simulink model "PTTransmCU"  (R2022b)
settings: Solver=ode45  StartTime=0.0  StopTime=inf  RelTol=1e-3  EnableMultiTasking=on
libraries: simulink x2, CarMaker4SL x1
(part 4 of 5)

== system PTTransmCU/CarMaker/IPG Vehicle/PowerTrain/TCU Example/PTTransmCU_In/CreateBus TCU GearboxIn8 ==
  In : Inport
  BusCreator : BusCreator  Inputs=23
  Demux : Demux  Outputs=23
      settings: DisplayOption=none
  Out : Outport  VectorParamsAs1DForOutWhenUnconnected=off
  wires:
  Demux/23 -> BusCreator/23  "TCU GearboxIn8 Clutch_dis i_TrqIn2Out"
  Demux/22 -> BusCreator/22  "TCU GearboxIn8 Clutch_dis Trq_out_trg"
  Demux/21 -> BusCreator/21  "TCU GearboxIn8 Clutch_dis Trq_out"
  Demux/20 -> BusCreator/20  "TCU GearboxIn8 Clutch_dis Trq_in"
  Demux/19 -> BusCreator/19  "TCU GearboxIn8 Clutch_dis rotv_out_trg"
  Demux/18 -> BusCreator/18  "TCU GearboxIn8 Clutch_dis rotv_out"
  Demux/17 -> BusCreator/17  "TCU GearboxIn8 Clutch_dis rotv_in"
  Demux/16 -> BusCreator/16  "TCU GearboxIn8 Clutch i_TrqIn2Out"
  Demux/15 -> BusCreator/15  "TCU GearboxIn8 Clutch Trq_out_trg"
  Demux/14 -> BusCreator/14  "TCU GearboxIn8 Clutch Trq_out"
  Demux/13 -> BusCreator/13  "TCU GearboxIn8 Clutch Trq_in"
  Demux/12 -> BusCreator/12  "TCU GearboxIn8 Clutch rotv_out_trg"
  Demux/11 -> BusCreator/11  "TCU GearboxIn8 Clutch rotv_out"
  Demux/10 -> BusCreator/10  "TCU GearboxIn8 Clutch rotv_in"
  Demux/9 -> BusCreator/9  "TCU GearboxIn8 Trq_out_trg"
  Demux/8 -> BusCreator/8  "TCU GearboxIn8 Trq_out"
  Demux/7 -> BusCreator/7  "TCU GearboxIn8 Trq_in"
  Demux/6 -> BusCreator/6  "TCU GearboxIn8 rotv_out"
  Demux/5 -> BusCreator/5  "TCU GearboxIn8 rotv_in_trg"
  Demux/4 -> BusCreator/4  "TCU GearboxIn8 rotv_in"
  Demux/3 -> BusCreator/3  "TCU GearboxIn8 i"
  Demux/2 -> BusCreator/2  "TCU GearboxIn8 GearNo_dis"
  Demux/1 -> BusCreator/1  "TCU GearboxIn8 GearNo"
  BusCreator/1 -> Out/1
  In/1 -> Demux/1

== system PTTransmCU/CarMaker/IPG Vehicle/PowerTrain/TCU Example/PTTransmCU_In/CreateBus TCU GearboxIn9 ==
  In : Inport
  BusCreator : BusCreator  Inputs=23
  Demux : Demux  Outputs=23
      settings: DisplayOption=none
  Out : Outport  VectorParamsAs1DForOutWhenUnconnected=off
  wires:
  Demux/23 -> BusCreator/23  "TCU GearboxIn9 Clutch_dis i_TrqIn2Out"
  Demux/22 -> BusCreator/22  "TCU GearboxIn9 Clutch_dis Trq_out_trg"
  Demux/21 -> BusCreator/21  "TCU GearboxIn9 Clutch_dis Trq_out"
  Demux/20 -> BusCreator/20  "TCU GearboxIn9 Clutch_dis Trq_in"
  Demux/19 -> BusCreator/19  "TCU GearboxIn9 Clutch_dis rotv_out_trg"
  Demux/18 -> BusCreator/18  "TCU GearboxIn9 Clutch_dis rotv_out"
  Demux/17 -> BusCreator/17  "TCU GearboxIn9 Clutch_dis rotv_in"
  Demux/16 -> BusCreator/16  "TCU GearboxIn9 Clutch i_TrqIn2Out"
  Demux/15 -> BusCreator/15  "TCU GearboxIn9 Clutch Trq_out_trg"
  Demux/14 -> BusCreator/14  "TCU GearboxIn9 Clutch Trq_out"
  Demux/13 -> BusCreator/13  "TCU GearboxIn9 Clutch Trq_in"
  Demux/12 -> BusCreator/12  "TCU GearboxIn9 Clutch rotv_out_trg"
  Demux/11 -> BusCreator/11  "TCU GearboxIn9 Clutch rotv_out"
  Demux/10 -> BusCreator/10  "TCU GearboxIn9 Clutch rotv_in"
  Demux/9 -> BusCreator/9  "TCU GearboxIn9 Trq_out_trg"
  Demux/8 -> BusCreator/8  "TCU GearboxIn9 Trq_out"
  Demux/7 -> BusCreator/7  "TCU GearboxIn9 Trq_in"
  Demux/6 -> BusCreator/6  "TCU GearboxIn9 rotv_out"
  Demux/5 -> BusCreator/5  "TCU GearboxIn9 rotv_in_trg"
  Demux/4 -> BusCreator/4  "TCU GearboxIn9 rotv_in"
  Demux/3 -> BusCreator/3  "TCU GearboxIn9 i"
  Demux/2 -> BusCreator/2  "TCU GearboxIn9 GearNo_dis"
  Demux/1 -> BusCreator/1  "TCU GearboxIn9 GearNo"
  BusCreator/1 -> Out/1
  In/1 -> Demux/1

== system PTTransmCU/CarMaker/IPG Vehicle/PowerTrain/TCU Example/PTTransmCU_In/CreateBus TCU GearboxOut0 ==
  In : Inport
  BusCreator : BusCreator  Inputs=6
  Demux : Demux  Outputs=6
      settings: DisplayOption=none
  Out : Outport  VectorParamsAs1DForOutWhenUnconnected=off
  wires:
  Demux/6 -> BusCreator/6  "TCU GearboxOut0 Clutch_dis Pos"
  Demux/5 -> BusCreator/5  "TCU GearboxOut0 Clutch Pos"
  Demux/4 -> BusCreator/4  "TCU GearboxOut0 i_trg"
  Demux/3 -> BusCreator/3  "TCU GearboxOut0 set_ParkBrake"
  Demux/2 -> BusCreator/2  "TCU GearboxOut0 GearNoTrg_dis"
  Demux/1 -> BusCreator/1  "TCU GearboxOut0 GearNoTrg"
  BusCreator/1 -> Out/1
  In/1 -> Demux/1

== system PTTransmCU/CarMaker/IPG Vehicle/PowerTrain/TCU Example/PTTransmCU_In/CreateBus TCU GearboxOut1 ==
  In : Inport
  BusCreator : BusCreator  Inputs=6
  Demux : Demux  Outputs=6
      settings: DisplayOption=none
  Out : Outport  VectorParamsAs1DForOutWhenUnconnected=off
  wires:
  Demux/6 -> BusCreator/6  "TCU GearboxOut1 Clutch_dis Pos"
  Demux/5 -> BusCreator/5  "TCU GearboxOut1 Clutch Pos"
  Demux/4 -> BusCreator/4  "TCU GearboxOut1 i_trg"
  Demux/3 -> BusCreator/3  "TCU GearboxOut1 set_ParkBrake"
  Demux/2 -> BusCreator/2  "TCU GearboxOut1 GearNoTrg_dis"
  Demux/1 -> BusCreator/1  "TCU GearboxOut1 GearNoTrg"
  BusCreator/1 -> Out/1
  In/1 -> Demux/1

== system PTTransmCU/CarMaker/IPG Vehicle/PowerTrain/TCU Example/PTTransmCU_In/CreateBus TCU GearboxOut10 ==
  In : Inport
  BusCreator : BusCreator  Inputs=6
  Demux : Demux  Outputs=6
      settings: DisplayOption=none
  Out : Outport  VectorParamsAs1DForOutWhenUnconnected=off
  wires:
  Demux/6 -> BusCreator/6  "TCU GearboxOut10 Clutch_dis Pos"
  Demux/5 -> BusCreator/5  "TCU GearboxOut10 Clutch Pos"
  Demux/4 -> BusCreator/4  "TCU GearboxOut10 i_trg"
  Demux/3 -> BusCreator/3  "TCU GearboxOut10 set_ParkBrake"
  Demux/2 -> BusCreator/2  "TCU GearboxOut10 GearNoTrg_dis"
  Demux/1 -> BusCreator/1  "TCU GearboxOut10 GearNoTrg"
  BusCreator/1 -> Out/1
  In/1 -> Demux/1

== system PTTransmCU/CarMaker/IPG Vehicle/PowerTrain/TCU Example/PTTransmCU_In/CreateBus TCU GearboxOut11 ==
  In : Inport
  BusCreator : BusCreator  Inputs=6
  Demux : Demux  Outputs=6
      settings: DisplayOption=none
  Out : Outport  VectorParamsAs1DForOutWhenUnconnected=off
  wires:
  Demux/6 -> BusCreator/6  "TCU GearboxOut11 Clutch_dis Pos"
  Demux/5 -> BusCreator/5  "TCU GearboxOut11 Clutch Pos"
  Demux/4 -> BusCreator/4  "TCU GearboxOut11 i_trg"
  Demux/3 -> BusCreator/3  "TCU GearboxOut11 set_ParkBrake"
  Demux/2 -> BusCreator/2  "TCU GearboxOut11 GearNoTrg_dis"
  Demux/1 -> BusCreator/1  "TCU GearboxOut11 GearNoTrg"
  BusCreator/1 -> Out/1
  In/1 -> Demux/1

== system PTTransmCU/CarMaker/IPG Vehicle/PowerTrain/TCU Example/PTTransmCU_In/CreateBus TCU GearboxOut2 ==
  In : Inport
  BusCreator : BusCreator  Inputs=6
  Demux : Demux  Outputs=6
      settings: DisplayOption=none
  Out : Outport  VectorParamsAs1DForOutWhenUnconnected=off
  wires:
  Demux/6 -> BusCreator/6  "TCU GearboxOut2 Clutch_dis Pos"
  Demux/5 -> BusCreator/5  "TCU GearboxOut2 Clutch Pos"
  Demux/4 -> BusCreator/4  "TCU GearboxOut2 i_trg"
  Demux/3 -> BusCreator/3  "TCU GearboxOut2 set_ParkBrake"
  Demux/2 -> BusCreator/2  "TCU GearboxOut2 GearNoTrg_dis"
  Demux/1 -> BusCreator/1  "TCU GearboxOut2 GearNoTrg"
  BusCreator/1 -> Out/1
  In/1 -> Demux/1

== system PTTransmCU/CarMaker/IPG Vehicle/PowerTrain/TCU Example/PTTransmCU_In/CreateBus TCU GearboxOut3 ==
  In : Inport
  BusCreator : BusCreator  Inputs=6
  Demux : Demux  Outputs=6
      settings: DisplayOption=none
  Out : Outport  VectorParamsAs1DForOutWhenUnconnected=off
  wires:
  Demux/6 -> BusCreator/6  "TCU GearboxOut3 Clutch_dis Pos"
  Demux/5 -> BusCreator/5  "TCU GearboxOut3 Clutch Pos"
  Demux/4 -> BusCreator/4  "TCU GearboxOut3 i_trg"
  Demux/3 -> BusCreator/3  "TCU GearboxOut3 set_ParkBrake"
  Demux/2 -> BusCreator/2  "TCU GearboxOut3 GearNoTrg_dis"
  Demux/1 -> BusCreator/1  "TCU GearboxOut3 GearNoTrg"
  BusCreator/1 -> Out/1
  In/1 -> Demux/1

== system PTTransmCU/CarMaker/IPG Vehicle/PowerTrain/TCU Example/PTTransmCU_In/CreateBus TCU GearboxOut4 ==
  In : Inport
  BusCreator : BusCreator  Inputs=6
  Demux : Demux  Outputs=6
      settings: DisplayOption=none
  Out : Outport  VectorParamsAs1DForOutWhenUnconnected=off
  wires:
  Demux/6 -> BusCreator/6  "TCU GearboxOut4 Clutch_dis Pos"
  Demux/5 -> BusCreator/5  "TCU GearboxOut4 Clutch Pos"
  Demux/4 -> BusCreator/4  "TCU GearboxOut4 i_trg"
  Demux/3 -> BusCreator/3  "TCU GearboxOut4 set_ParkBrake"
  Demux/2 -> BusCreator/2  "TCU GearboxOut4 GearNoTrg_dis"
  Demux/1 -> BusCreator/1  "TCU GearboxOut4 GearNoTrg"
  BusCreator/1 -> Out/1
  In/1 -> Demux/1

== system PTTransmCU/CarMaker/IPG Vehicle/PowerTrain/TCU Example/PTTransmCU_In/CreateBus TCU GearboxOut5 ==
  In : Inport
  BusCreator : BusCreator  Inputs=6
  Demux : Demux  Outputs=6
      settings: DisplayOption=none
  Out : Outport  VectorParamsAs1DForOutWhenUnconnected=off
  wires:
  Demux/6 -> BusCreator/6  "TCU GearboxOut5 Clutch_dis Pos"
  Demux/5 -> BusCreator/5  "TCU GearboxOut5 Clutch Pos"
  Demux/4 -> BusCreator/4  "TCU GearboxOut5 i_trg"
  Demux/3 -> BusCreator/3  "TCU GearboxOut5 set_ParkBrake"
  Demux/2 -> BusCreator/2  "TCU GearboxOut5 GearNoTrg_dis"
  Demux/1 -> BusCreator/1  "TCU GearboxOut5 GearNoTrg"
  BusCreator/1 -> Out/1
  In/1 -> Demux/1

== system PTTransmCU/CarMaker/IPG Vehicle/PowerTrain/TCU Example/PTTransmCU_In/CreateBus TCU GearboxOut6 ==
  In : Inport
  BusCreator : BusCreator  Inputs=6
  Demux : Demux  Outputs=6
      settings: DisplayOption=none
  Out : Outport  VectorParamsAs1DForOutWhenUnconnected=off
  wires:
  Demux/6 -> BusCreator/6  "TCU GearboxOut6 Clutch_dis Pos"
  Demux/5 -> BusCreator/5  "TCU GearboxOut6 Clutch Pos"
  Demux/4 -> BusCreator/4  "TCU GearboxOut6 i_trg"
  Demux/3 -> BusCreator/3  "TCU GearboxOut6 set_ParkBrake"
  Demux/2 -> BusCreator/2  "TCU GearboxOut6 GearNoTrg_dis"
  Demux/1 -> BusCreator/1  "TCU GearboxOut6 GearNoTrg"
  BusCreator/1 -> Out/1
  In/1 -> Demux/1

== system PTTransmCU/CarMaker/IPG Vehicle/PowerTrain/TCU Example/PTTransmCU_In/CreateBus TCU GearboxOut7 ==
  In : Inport
  BusCreator : BusCreator  Inputs=6
  Demux : Demux  Outputs=6
      settings: DisplayOption=none
  Out : Outport  VectorParamsAs1DForOutWhenUnconnected=off
  wires:
  Demux/6 -> BusCreator/6  "TCU GearboxOut7 Clutch_dis Pos"
  Demux/5 -> BusCreator/5  "TCU GearboxOut7 Clutch Pos"
  Demux/4 -> BusCreator/4  "TCU GearboxOut7 i_trg"
  Demux/3 -> BusCreator/3  "TCU GearboxOut7 set_ParkBrake"
  Demux/2 -> BusCreator/2  "TCU GearboxOut7 GearNoTrg_dis"
  Demux/1 -> BusCreator/1  "TCU GearboxOut7 GearNoTrg"
  BusCreator/1 -> Out/1
  In/1 -> Demux/1

== system PTTransmCU/CarMaker/IPG Vehicle/PowerTrain/TCU Example/PTTransmCU_In/CreateBus TCU GearboxOut8 ==
  In : Inport
  BusCreator : BusCreator  Inputs=6
  Demux : Demux  Outputs=6
      settings: DisplayOption=none
  Out : Outport  VectorParamsAs1DForOutWhenUnconnected=off
  wires:
  Demux/6 -> BusCreator/6  "TCU GearboxOut8 Clutch_dis Pos"
  Demux/5 -> BusCreator/5  "TCU GearboxOut8 Clutch Pos"
  Demux/4 -> BusCreator/4  "TCU GearboxOut8 i_trg"
  Demux/3 -> BusCreator/3  "TCU GearboxOut8 set_ParkBrake"
  Demux/2 -> BusCreator/2  "TCU GearboxOut8 GearNoTrg_dis"
  Demux/1 -> BusCreator/1  "TCU GearboxOut8 GearNoTrg"
  BusCreator/1 -> Out/1
  In/1 -> Demux/1

== system PTTransmCU/CarMaker/IPG Vehicle/PowerTrain/TCU Example/PTTransmCU_In/CreateBus TCU GearboxOut9 ==
  In : Inport
  BusCreator : BusCreator  Inputs=6
  Demux : Demux  Outputs=6
      settings: DisplayOption=none
  Out : Outport  VectorParamsAs1DForOutWhenUnconnected=off
  wires:
  Demux/6 -> BusCreator/6  "TCU GearboxOut9 Clutch_dis Pos"
  Demux/5 -> BusCreator/5  "TCU GearboxOut9 Clutch Pos"
  Demux/4 -> BusCreator/4  "TCU GearboxOut9 i_trg"
  Demux/3 -> BusCreator/3  "TCU GearboxOut9 set_ParkBrake"
  Demux/2 -> BusCreator/2  "TCU GearboxOut9 GearNoTrg_dis"
  Demux/1 -> BusCreator/1  "TCU GearboxOut9 GearNoTrg"
  BusCreator/1 -> Out/1
  In/1 -> Demux/1

== system PTTransmCU/CarMaker/IPG Vehicle/PowerTrain/TCU Example/PTTransmCU_In/CreateBus TCU Input ==
  In : Inport
  BusCreator : BusCreator  Inputs=3
  Demux : Demux  Outputs=3
      settings: DisplayOption=none
  Out : Outport  VectorParamsAs1DForOutWhenUnconnected=off
  wires:
  Demux/3 -> BusCreator/3  "TCU SelectorCtrl"
  Demux/2 -> BusCreator/2  "TCU Load"
  Demux/1 -> BusCreator/1  "TCU Ignition"
  BusCreator/1 -> Out/1
  In/1 -> Demux/1

== system PTTransmCU/CarMaker/IPG Vehicle/PowerTrain/TCU Example/PTTransmCU_In/CreateBus TCU_Cfg Gearbox0 ==
  In : Inport
  BusCreator : BusCreator  Inputs=38
  Demux : Demux  Outputs=38
      settings: DisplayOption=none
  Out : Outport  VectorParamsAs1DForOutWhenUnconnected=off
  wires:
  Demux/38 -> BusCreator/38  "TCU_Cfg Gearbox0 iBGear16"
  Demux/37 -> BusCreator/37  "TCU_Cfg Gearbox0 iBGear15"
  Demux/36 -> BusCreator/36  "TCU_Cfg Gearbox0 iBGear14"
  Demux/35 -> BusCreator/35  "TCU_Cfg Gearbox0 iBGear13"
  Demux/34 -> BusCreator/34  "TCU_Cfg Gearbox0 iBGear12"
  Demux/33 -> BusCreator/33  "TCU_Cfg Gearbox0 iBGear11"
  Demux/32 -> BusCreator/32  "TCU_Cfg Gearbox0 iBGear10"
  Demux/31 -> BusCreator/31  "TCU_Cfg Gearbox0 iBGear9"
  Demux/30 -> BusCreator/30  "TCU_Cfg Gearbox0 iBGear8"
  Demux/29 -> BusCreator/29  "TCU_Cfg Gearbox0 iBGear7"
  Demux/28 -> BusCreator/28  "TCU_Cfg Gearbox0 iBGear6"
  Demux/27 -> BusCreator/27  "TCU_Cfg Gearbox0 iBGear5"
  Demux/26 -> BusCreator/26  "TCU_Cfg Gearbox0 iBGear4"
  Demux/25 -> BusCreator/25  "TCU_Cfg Gearbox0 iBGear3"
  Demux/24 -> BusCreator/24  "TCU_Cfg Gearbox0 iBGear2"
  Demux/23 -> BusCreator/23  "TCU_Cfg Gearbox0 iBGear1"
  Demux/22 -> BusCreator/22  "TCU_Cfg Gearbox0 iBGear0"
  Demux/21 -> BusCreator/21  "TCU_Cfg Gearbox0 nBGears"
  Demux/20 -> BusCreator/20  "TCU_Cfg Gearbox0 iFGear16"
  Demux/19 -> BusCreator/19  "TCU_Cfg Gearbox0 iFGear15"
  Demux/18 -> BusCreator/18  "TCU_Cfg Gearbox0 iFGear14"
  Demux/17 -> BusCreator/17  "TCU_Cfg Gearbox0 iFGear13"
  Demux/16 -> BusCreator/16  "TCU_Cfg Gearbox0 iFGear12"
  Demux/15 -> BusCreator/15  "TCU_Cfg Gearbox0 iFGear11"
  Demux/14 -> BusCreator/14  "TCU_Cfg Gearbox0 iFGear10"
  Demux/13 -> BusCreator/13  "TCU_Cfg Gearbox0 iFGear9"
  Demux/12 -> BusCreator/12  "TCU_Cfg Gearbox0 iFGear8"
  Demux/11 -> BusCreator/11  "TCU_Cfg Gearbox0 iFGear7"
  Demux/10 -> BusCreator/10  "TCU_Cfg Gearbox0 iFGear6"
  Demux/9 -> BusCreator/9  "TCU_Cfg Gearbox0 iFGear5"
  Demux/8 -> BusCreator/8  "TCU_Cfg Gearbox0 iFGear4"
  Demux/7 -> BusCreator/7  "TCU_Cfg Gearbox0 iFGear3"
  Demux/6 -> BusCreator/6  "TCU_Cfg Gearbox0 iFGear2"
  Demux/5 -> BusCreator/5  "TCU_Cfg Gearbox0 iFGear1"
  Demux/4 -> BusCreator/4  "TCU_Cfg Gearbox0 iFGear0"
  Demux/3 -> BusCreator/3  "TCU_Cfg Gearbox0 nFGears"
  Demux/2 -> BusCreator/2  "TCU_Cfg Gearbox0 ClKind"
  Demux/1 -> BusCreator/1  "TCU_Cfg Gearbox0 GBKind"
  BusCreator/1 -> Out/1
  In/1 -> Demux/1

== system PTTransmCU/CarMaker/IPG Vehicle/PowerTrain/TCU Example/PTTransmCU_In/CreateBus TCU_Cfg Gearbox1 ==
  In : Inport
  BusCreator : BusCreator  Inputs=38
  Demux : Demux  Outputs=38
      settings: DisplayOption=none
  Out : Outport  VectorParamsAs1DForOutWhenUnconnected=off
  wires:
  Demux/38 -> BusCreator/38  "TCU_Cfg Gearbox1 iBGear16"
  Demux/37 -> BusCreator/37  "TCU_Cfg Gearbox1 iBGear15"
  Demux/36 -> BusCreator/36  "TCU_Cfg Gearbox1 iBGear14"
  Demux/35 -> BusCreator/35  "TCU_Cfg Gearbox1 iBGear13"
  Demux/34 -> BusCreator/34  "TCU_Cfg Gearbox1 iBGear12"
  Demux/33 -> BusCreator/33  "TCU_Cfg Gearbox1 iBGear11"
  Demux/32 -> BusCreator/32  "TCU_Cfg Gearbox1 iBGear10"
  Demux/31 -> BusCreator/31  "TCU_Cfg Gearbox1 iBGear9"
  Demux/30 -> BusCreator/30  "TCU_Cfg Gearbox1 iBGear8"
  Demux/29 -> BusCreator/29  "TCU_Cfg Gearbox1 iBGear7"
  Demux/28 -> BusCreator/28  "TCU_Cfg Gearbox1 iBGear6"
  Demux/27 -> BusCreator/27  "TCU_Cfg Gearbox1 iBGear5"
  Demux/26 -> BusCreator/26  "TCU_Cfg Gearbox1 iBGear4"
  Demux/25 -> BusCreator/25  "TCU_Cfg Gearbox1 iBGear3"
  Demux/24 -> BusCreator/24  "TCU_Cfg Gearbox1 iBGear2"
  Demux/23 -> BusCreator/23  "TCU_Cfg Gearbox1 iBGear1"
  Demux/22 -> BusCreator/22  "TCU_Cfg Gearbox1 iBGear0"
  Demux/21 -> BusCreator/21  "TCU_Cfg Gearbox1 nBGears"
  Demux/20 -> BusCreator/20  "TCU_Cfg Gearbox1 iFGear16"
  Demux/19 -> BusCreator/19  "TCU_Cfg Gearbox1 iFGear15"
  Demux/18 -> BusCreator/18  "TCU_Cfg Gearbox1 iFGear14"
  Demux/17 -> BusCreator/17  "TCU_Cfg Gearbox1 iFGear13"
  Demux/16 -> BusCreator/16  "TCU_Cfg Gearbox1 iFGear12"
  Demux/15 -> BusCreator/15  "TCU_Cfg Gearbox1 iFGear11"
  Demux/14 -> BusCreator/14  "TCU_Cfg Gearbox1 iFGear10"
  Demux/13 -> BusCreator/13  "TCU_Cfg Gearbox1 iFGear9"
  Demux/12 -> BusCreator/12  "TCU_Cfg Gearbox1 iFGear8"
  Demux/11 -> BusCreator/11  "TCU_Cfg Gearbox1 iFGear7"
  Demux/10 -> BusCreator/10  "TCU_Cfg Gearbox1 iFGear6"
  Demux/9 -> BusCreator/9  "TCU_Cfg Gearbox1 iFGear5"
  Demux/8 -> BusCreator/8  "TCU_Cfg Gearbox1 iFGear4"
  Demux/7 -> BusCreator/7  "TCU_Cfg Gearbox1 iFGear3"
  Demux/6 -> BusCreator/6  "TCU_Cfg Gearbox1 iFGear2"
  Demux/5 -> BusCreator/5  "TCU_Cfg Gearbox1 iFGear1"
  Demux/4 -> BusCreator/4  "TCU_Cfg Gearbox1 iFGear0"
  Demux/3 -> BusCreator/3  "TCU_Cfg Gearbox1 nFGears"
  Demux/2 -> BusCreator/2  "TCU_Cfg Gearbox1 ClKind"
  Demux/1 -> BusCreator/1  "TCU_Cfg Gearbox1 GBKind"
  BusCreator/1 -> Out/1
  In/1 -> Demux/1

== system PTTransmCU/CarMaker/IPG Vehicle/PowerTrain/TCU Example/PTTransmCU_In/CreateBus TCU_Cfg Gearbox10 ==
  In : Inport
  BusCreator : BusCreator  Inputs=38
  Demux : Demux  Outputs=38
      settings: DisplayOption=none
  Out : Outport  VectorParamsAs1DForOutWhenUnconnected=off
  wires:
  Demux/38 -> BusCreator/38  "TCU_Cfg Gearbox10 iBGear16"
  Demux/37 -> BusCreator/37  "TCU_Cfg Gearbox10 iBGear15"
  Demux/36 -> BusCreator/36  "TCU_Cfg Gearbox10 iBGear14"
  Demux/35 -> BusCreator/35  "TCU_Cfg Gearbox10 iBGear13"
  Demux/34 -> BusCreator/34  "TCU_Cfg Gearbox10 iBGear12"
  Demux/33 -> BusCreator/33  "TCU_Cfg Gearbox10 iBGear11"
  Demux/32 -> BusCreator/32  "TCU_Cfg Gearbox10 iBGear10"
  Demux/31 -> BusCreator/31  "TCU_Cfg Gearbox10 iBGear9"
  Demux/30 -> BusCreator/30  "TCU_Cfg Gearbox10 iBGear8"
  Demux/29 -> BusCreator/29  "TCU_Cfg Gearbox10 iBGear7"
  Demux/28 -> BusCreator/28  "TCU_Cfg Gearbox10 iBGear6"
  Demux/27 -> BusCreator/27  "TCU_Cfg Gearbox10 iBGear5"
  Demux/26 -> BusCreator/26  "TCU_Cfg Gearbox10 iBGear4"
  Demux/25 -> BusCreator/25  "TCU_Cfg Gearbox10 iBGear3"
  Demux/24 -> BusCreator/24  "TCU_Cfg Gearbox10 iBGear2"
  Demux/23 -> BusCreator/23  "TCU_Cfg Gearbox10 iBGear1"
  Demux/22 -> BusCreator/22  "TCU_Cfg Gearbox10 iBGear0"
  Demux/21 -> BusCreator/21  "TCU_Cfg Gearbox10 nBGears"
  Demux/20 -> BusCreator/20  "TCU_Cfg Gearbox10 iFGear16"
  Demux/19 -> BusCreator/19  "TCU_Cfg Gearbox10 iFGear15"
  Demux/18 -> BusCreator/18  "TCU_Cfg Gearbox10 iFGear14"
  Demux/17 -> BusCreator/17  "TCU_Cfg Gearbox10 iFGear13"
  Demux/16 -> BusCreator/16  "TCU_Cfg Gearbox10 iFGear12"
  Demux/15 -> BusCreator/15  "TCU_Cfg Gearbox10 iFGear11"
  Demux/14 -> BusCreator/14  "TCU_Cfg Gearbox10 iFGear10"
  Demux/13 -> BusCreator/13  "TCU_Cfg Gearbox10 iFGear9"
  Demux/12 -> BusCreator/12  "TCU_Cfg Gearbox10 iFGear8"
  Demux/11 -> BusCreator/11  "TCU_Cfg Gearbox10 iFGear7"
  Demux/10 -> BusCreator/10  "TCU_Cfg Gearbox10 iFGear6"
  Demux/9 -> BusCreator/9  "TCU_Cfg Gearbox10 iFGear5"
  Demux/8 -> BusCreator/8  "TCU_Cfg Gearbox10 iFGear4"
  Demux/7 -> BusCreator/7  "TCU_Cfg Gearbox10 iFGear3"
  Demux/6 -> BusCreator/6  "TCU_Cfg Gearbox10 iFGear2"
  Demux/5 -> BusCreator/5  "TCU_Cfg Gearbox10 iFGear1"
  Demux/4 -> BusCreator/4  "TCU_Cfg Gearbox10 iFGear0"
  Demux/3 -> BusCreator/3  "TCU_Cfg Gearbox10 nFGears"
  Demux/2 -> BusCreator/2  "TCU_Cfg Gearbox10 ClKind"
  Demux/1 -> BusCreator/1  "TCU_Cfg Gearbox10 GBKind"
  BusCreator/1 -> Out/1
  In/1 -> Demux/1

== system PTTransmCU/CarMaker/IPG Vehicle/PowerTrain/TCU Example/PTTransmCU_In/CreateBus TCU_Cfg Gearbox11 ==
  In : Inport
  BusCreator : BusCreator  Inputs=38
  Demux : Demux  Outputs=38
      settings: DisplayOption=none
  Out : Outport  VectorParamsAs1DForOutWhenUnconnected=off
  wires:
  Demux/38 -> BusCreator/38  "TCU_Cfg Gearbox11 iBGear16"
  Demux/37 -> BusCreator/37  "TCU_Cfg Gearbox11 iBGear15"
  Demux/36 -> BusCreator/36  "TCU_Cfg Gearbox11 iBGear14"
  Demux/35 -> BusCreator/35  "TCU_Cfg Gearbox11 iBGear13"
  Demux/34 -> BusCreator/34  "TCU_Cfg Gearbox11 iBGear12"
  Demux/33 -> BusCreator/33  "TCU_Cfg Gearbox11 iBGear11"
  Demux/32 -> BusCreator/32  "TCU_Cfg Gearbox11 iBGear10"
  Demux/31 -> BusCreator/31  "TCU_Cfg Gearbox11 iBGear9"
  Demux/30 -> BusCreator/30  "TCU_Cfg Gearbox11 iBGear8"
  Demux/29 -> BusCreator/29  "TCU_Cfg Gearbox11 iBGear7"
  Demux/28 -> BusCreator/28  "TCU_Cfg Gearbox11 iBGear6"
  Demux/27 -> BusCreator/27  "TCU_Cfg Gearbox11 iBGear5"
  Demux/26 -> BusCreator/26  "TCU_Cfg Gearbox11 iBGear4"
  Demux/25 -> BusCreator/25  "TCU_Cfg Gearbox11 iBGear3"
  Demux/24 -> BusCreator/24  "TCU_Cfg Gearbox11 iBGear2"
  Demux/23 -> BusCreator/23  "TCU_Cfg Gearbox11 iBGear1"
  Demux/22 -> BusCreator/22  "TCU_Cfg Gearbox11 iBGear0"
  Demux/21 -> BusCreator/21  "TCU_Cfg Gearbox11 nBGears"
  Demux/20 -> BusCreator/20  "TCU_Cfg Gearbox11 iFGear16"
  Demux/19 -> BusCreator/19  "TCU_Cfg Gearbox11 iFGear15"
  Demux/18 -> BusCreator/18  "TCU_Cfg Gearbox11 iFGear14"
  Demux/17 -> BusCreator/17  "TCU_Cfg Gearbox11 iFGear13"
  Demux/16 -> BusCreator/16  "TCU_Cfg Gearbox11 iFGear12"
  Demux/15 -> BusCreator/15  "TCU_Cfg Gearbox11 iFGear11"
  Demux/14 -> BusCreator/14  "TCU_Cfg Gearbox11 iFGear10"
  Demux/13 -> BusCreator/13  "TCU_Cfg Gearbox11 iFGear9"
  Demux/12 -> BusCreator/12  "TCU_Cfg Gearbox11 iFGear8"
  Demux/11 -> BusCreator/11  "TCU_Cfg Gearbox11 iFGear7"
  Demux/10 -> BusCreator/10  "TCU_Cfg Gearbox11 iFGear6"
  Demux/9 -> BusCreator/9  "TCU_Cfg Gearbox11 iFGear5"
  Demux/8 -> BusCreator/8  "TCU_Cfg Gearbox11 iFGear4"
  Demux/7 -> BusCreator/7  "TCU_Cfg Gearbox11 iFGear3"
  Demux/6 -> BusCreator/6  "TCU_Cfg Gearbox11 iFGear2"
  Demux/5 -> BusCreator/5  "TCU_Cfg Gearbox11 iFGear1"
  Demux/4 -> BusCreator/4  "TCU_Cfg Gearbox11 iFGear0"
  Demux/3 -> BusCreator/3  "TCU_Cfg Gearbox11 nFGears"
  Demux/2 -> BusCreator/2  "TCU_Cfg Gearbox11 ClKind"
  Demux/1 -> BusCreator/1  "TCU_Cfg Gearbox11 GBKind"
  BusCreator/1 -> Out/1
  In/1 -> Demux/1

== system PTTransmCU/CarMaker/IPG Vehicle/PowerTrain/TCU Example/PTTransmCU_In/CreateBus TCU_Cfg Gearbox2 ==
  In : Inport
  BusCreator : BusCreator  Inputs=38
  Demux : Demux  Outputs=38
      settings: DisplayOption=none
  Out : Outport  VectorParamsAs1DForOutWhenUnconnected=off
  wires:
  Demux/38 -> BusCreator/38  "TCU_Cfg Gearbox2 iBGear16"
  Demux/37 -> BusCreator/37  "TCU_Cfg Gearbox2 iBGear15"
  Demux/36 -> BusCreator/36  "TCU_Cfg Gearbox2 iBGear14"
  Demux/35 -> BusCreator/35  "TCU_Cfg Gearbox2 iBGear13"
  Demux/34 -> BusCreator/34  "TCU_Cfg Gearbox2 iBGear12"
  Demux/33 -> BusCreator/33  "TCU_Cfg Gearbox2 iBGear11"
  Demux/32 -> BusCreator/32  "TCU_Cfg Gearbox2 iBGear10"
  Demux/31 -> BusCreator/31  "TCU_Cfg Gearbox2 iBGear9"
  Demux/30 -> BusCreator/30  "TCU_Cfg Gearbox2 iBGear8"
  Demux/29 -> BusCreator/29  "TCU_Cfg Gearbox2 iBGear7"
  Demux/28 -> BusCreator/28  "TCU_Cfg Gearbox2 iBGear6"
  Demux/27 -> BusCreator/27  "TCU_Cfg Gearbox2 iBGear5"
  Demux/26 -> BusCreator/26  "TCU_Cfg Gearbox2 iBGear4"
  Demux/25 -> BusCreator/25  "TCU_Cfg Gearbox2 iBGear3"
  Demux/24 -> BusCreator/24  "TCU_Cfg Gearbox2 iBGear2"
  Demux/23 -> BusCreator/23  "TCU_Cfg Gearbox2 iBGear1"
  Demux/22 -> BusCreator/22  "TCU_Cfg Gearbox2 iBGear0"
  Demux/21 -> BusCreator/21  "TCU_Cfg Gearbox2 nBGears"
  Demux/20 -> BusCreator/20  "TCU_Cfg Gearbox2 iFGear16"
  Demux/19 -> BusCreator/19  "TCU_Cfg Gearbox2 iFGear15"
  Demux/18 -> BusCreator/18  "TCU_Cfg Gearbox2 iFGear14"
  Demux/17 -> BusCreator/17  "TCU_Cfg Gearbox2 iFGear13"
  Demux/16 -> BusCreator/16  "TCU_Cfg Gearbox2 iFGear12"
  Demux/15 -> BusCreator/15  "TCU_Cfg Gearbox2 iFGear11"
  Demux/14 -> BusCreator/14  "TCU_Cfg Gearbox2 iFGear10"
  Demux/13 -> BusCreator/13  "TCU_Cfg Gearbox2 iFGear9"
  Demux/12 -> BusCreator/12  "TCU_Cfg Gearbox2 iFGear8"
  Demux/11 -> BusCreator/11  "TCU_Cfg Gearbox2 iFGear7"
  Demux/10 -> BusCreator/10  "TCU_Cfg Gearbox2 iFGear6"
  Demux/9 -> BusCreator/9  "TCU_Cfg Gearbox2 iFGear5"
  Demux/8 -> BusCreator/8  "TCU_Cfg Gearbox2 iFGear4"
  Demux/7 -> BusCreator/7  "TCU_Cfg Gearbox2 iFGear3"
  Demux/6 -> BusCreator/6  "TCU_Cfg Gearbox2 iFGear2"
  Demux/5 -> BusCreator/5  "TCU_Cfg Gearbox2 iFGear1"
  Demux/4 -> BusCreator/4  "TCU_Cfg Gearbox2 iFGear0"
  Demux/3 -> BusCreator/3  "TCU_Cfg Gearbox2 nFGears"
  Demux/2 -> BusCreator/2  "TCU_Cfg Gearbox2 ClKind"
  Demux/1 -> BusCreator/1  "TCU_Cfg Gearbox2 GBKind"
  BusCreator/1 -> Out/1
  In/1 -> Demux/1

== system PTTransmCU/CarMaker/IPG Vehicle/PowerTrain/TCU Example/PTTransmCU_In/CreateBus TCU_Cfg Gearbox3 ==
  In : Inport
  BusCreator : BusCreator  Inputs=38
  Demux : Demux  Outputs=38
      settings: DisplayOption=none
  Out : Outport  VectorParamsAs1DForOutWhenUnconnected=off
  wires:
  Demux/38 -> BusCreator/38  "TCU_Cfg Gearbox3 iBGear16"
  Demux/37 -> BusCreator/37  "TCU_Cfg Gearbox3 iBGear15"
  Demux/36 -> BusCreator/36  "TCU_Cfg Gearbox3 iBGear14"
  Demux/35 -> BusCreator/35  "TCU_Cfg Gearbox3 iBGear13"
  Demux/34 -> BusCreator/34  "TCU_Cfg Gearbox3 iBGear12"
  Demux/33 -> BusCreator/33  "TCU_Cfg Gearbox3 iBGear11"
  Demux/32 -> BusCreator/32  "TCU_Cfg Gearbox3 iBGear10"
  Demux/31 -> BusCreator/31  "TCU_Cfg Gearbox3 iBGear9"
  Demux/30 -> BusCreator/30  "TCU_Cfg Gearbox3 iBGear8"
  Demux/29 -> BusCreator/29  "TCU_Cfg Gearbox3 iBGear7"
  Demux/28 -> BusCreator/28  "TCU_Cfg Gearbox3 iBGear6"
  Demux/27 -> BusCreator/27  "TCU_Cfg Gearbox3 iBGear5"
  Demux/26 -> BusCreator/26  "TCU_Cfg Gearbox3 iBGear4"
  Demux/25 -> BusCreator/25  "TCU_Cfg Gearbox3 iBGear3"
  Demux/24 -> BusCreator/24  "TCU_Cfg Gearbox3 iBGear2"
  Demux/23 -> BusCreator/23  "TCU_Cfg Gearbox3 iBGear1"
  Demux/22 -> BusCreator/22  "TCU_Cfg Gearbox3 iBGear0"
  Demux/21 -> BusCreator/21  "TCU_Cfg Gearbox3 nBGears"
  Demux/20 -> BusCreator/20  "TCU_Cfg Gearbox3 iFGear16"
  Demux/19 -> BusCreator/19  "TCU_Cfg Gearbox3 iFGear15"
  Demux/18 -> BusCreator/18  "TCU_Cfg Gearbox3 iFGear14"
  Demux/17 -> BusCreator/17  "TCU_Cfg Gearbox3 iFGear13"
  Demux/16 -> BusCreator/16  "TCU_Cfg Gearbox3 iFGear12"
  Demux/15 -> BusCreator/15  "TCU_Cfg Gearbox3 iFGear11"
  Demux/14 -> BusCreator/14  "TCU_Cfg Gearbox3 iFGear10"
  Demux/13 -> BusCreator/13  "TCU_Cfg Gearbox3 iFGear9"
  Demux/12 -> BusCreator/12  "TCU_Cfg Gearbox3 iFGear8"
  Demux/11 -> BusCreator/11  "TCU_Cfg Gearbox3 iFGear7"
  Demux/10 -> BusCreator/10  "TCU_Cfg Gearbox3 iFGear6"
  Demux/9 -> BusCreator/9  "TCU_Cfg Gearbox3 iFGear5"
  Demux/8 -> BusCreator/8  "TCU_Cfg Gearbox3 iFGear4"
  Demux/7 -> BusCreator/7  "TCU_Cfg Gearbox3 iFGear3"
  Demux/6 -> BusCreator/6  "TCU_Cfg Gearbox3 iFGear2"
  Demux/5 -> BusCreator/5  "TCU_Cfg Gearbox3 iFGear1"
  Demux/4 -> BusCreator/4  "TCU_Cfg Gearbox3 iFGear0"
  Demux/3 -> BusCreator/3  "TCU_Cfg Gearbox3 nFGears"
  Demux/2 -> BusCreator/2  "TCU_Cfg Gearbox3 ClKind"
  Demux/1 -> BusCreator/1  "TCU_Cfg Gearbox3 GBKind"
  BusCreator/1 -> Out/1
  In/1 -> Demux/1

== system PTTransmCU/CarMaker/IPG Vehicle/PowerTrain/TCU Example/PTTransmCU_In/CreateBus TCU_Cfg Gearbox4 ==
  In : Inport
  BusCreator : BusCreator  Inputs=38
  Demux : Demux  Outputs=38
      settings: DisplayOption=none
  Out : Outport  VectorParamsAs1DForOutWhenUnconnected=off
  wires:
  Demux/38 -> BusCreator/38  "TCU_Cfg Gearbox4 iBGear16"
  Demux/37 -> BusCreator/37  "TCU_Cfg Gearbox4 iBGear15"
  Demux/36 -> BusCreator/36  "TCU_Cfg Gearbox4 iBGear14"
  Demux/35 -> BusCreator/35  "TCU_Cfg Gearbox4 iBGear13"
  Demux/34 -> BusCreator/34  "TCU_Cfg Gearbox4 iBGear12"
  Demux/33 -> BusCreator/33  "TCU_Cfg Gearbox4 iBGear11"
  Demux/32 -> BusCreator/32  "TCU_Cfg Gearbox4 iBGear10"
  Demux/31 -> BusCreator/31  "TCU_Cfg Gearbox4 iBGear9"
  Demux/30 -> BusCreator/30  "TCU_Cfg Gearbox4 iBGear8"
  Demux/29 -> BusCreator/29  "TCU_Cfg Gearbox4 iBGear7"
  Demux/28 -> BusCreator/28  "TCU_Cfg Gearbox4 iBGear6"
  Demux/27 -> BusCreator/27  "TCU_Cfg Gearbox4 iBGear5"
  Demux/26 -> BusCreator/26  "TCU_Cfg Gearbox4 iBGear4"
  Demux/25 -> BusCreator/25  "TCU_Cfg Gearbox4 iBGear3"
  Demux/24 -> BusCreator/24  "TCU_Cfg Gearbox4 iBGear2"
  Demux/23 -> BusCreator/23  "TCU_Cfg Gearbox4 iBGear1"
  Demux/22 -> BusCreator/22  "TCU_Cfg Gearbox4 iBGear0"
  Demux/21 -> BusCreator/21  "TCU_Cfg Gearbox4 nBGears"
  Demux/20 -> BusCreator/20  "TCU_Cfg Gearbox4 iFGear16"
  Demux/19 -> BusCreator/19  "TCU_Cfg Gearbox4 iFGear15"
  Demux/18 -> BusCreator/18  "TCU_Cfg Gearbox4 iFGear14"
  Demux/17 -> BusCreator/17  "TCU_Cfg Gearbox4 iFGear13"
  Demux/16 -> BusCreator/16  "TCU_Cfg Gearbox4 iFGear12"
  Demux/15 -> BusCreator/15  "TCU_Cfg Gearbox4 iFGear11"
  Demux/14 -> BusCreator/14  "TCU_Cfg Gearbox4 iFGear10"
  Demux/13 -> BusCreator/13  "TCU_Cfg Gearbox4 iFGear9"
  Demux/12 -> BusCreator/12  "TCU_Cfg Gearbox4 iFGear8"
  Demux/11 -> BusCreator/11  "TCU_Cfg Gearbox4 iFGear7"
  Demux/10 -> BusCreator/10  "TCU_Cfg Gearbox4 iFGear6"
  Demux/9 -> BusCreator/9  "TCU_Cfg Gearbox4 iFGear5"
  Demux/8 -> BusCreator/8  "TCU_Cfg Gearbox4 iFGear4"
  Demux/7 -> BusCreator/7  "TCU_Cfg Gearbox4 iFGear3"
  Demux/6 -> BusCreator/6  "TCU_Cfg Gearbox4 iFGear2"
  Demux/5 -> BusCreator/5  "TCU_Cfg Gearbox4 iFGear1"
  Demux/4 -> BusCreator/4  "TCU_Cfg Gearbox4 iFGear0"
  Demux/3 -> BusCreator/3  "TCU_Cfg Gearbox4 nFGears"
  Demux/2 -> BusCreator/2  "TCU_Cfg Gearbox4 ClKind"
  Demux/1 -> BusCreator/1  "TCU_Cfg Gearbox4 GBKind"
  BusCreator/1 -> Out/1
  In/1 -> Demux/1

== system PTTransmCU/CarMaker/IPG Vehicle/PowerTrain/TCU Example/PTTransmCU_In/CreateBus TCU_Cfg Gearbox5 ==
  In : Inport
  BusCreator : BusCreator  Inputs=38
  Demux : Demux  Outputs=38
      settings: DisplayOption=none
  Out : Outport  VectorParamsAs1DForOutWhenUnconnected=off
  wires:
  Demux/38 -> BusCreator/38  "TCU_Cfg Gearbox5 iBGear16"
  Demux/37 -> BusCreator/37  "TCU_Cfg Gearbox5 iBGear15"
  Demux/36 -> BusCreator/36  "TCU_Cfg Gearbox5 iBGear14"
  Demux/35 -> BusCreator/35  "TCU_Cfg Gearbox5 iBGear13"
  Demux/34 -> BusCreator/34  "TCU_Cfg Gearbox5 iBGear12"
  Demux/33 -> BusCreator/33  "TCU_Cfg Gearbox5 iBGear11"
  Demux/32 -> BusCreator/32  "TCU_Cfg Gearbox5 iBGear10"
  Demux/31 -> BusCreator/31  "TCU_Cfg Gearbox5 iBGear9"
  Demux/30 -> BusCreator/30  "TCU_Cfg Gearbox5 iBGear8"
  Demux/29 -> BusCreator/29  "TCU_Cfg Gearbox5 iBGear7"
  Demux/28 -> BusCreator/28  "TCU_Cfg Gearbox5 iBGear6"
  Demux/27 -> BusCreator/27  "TCU_Cfg Gearbox5 iBGear5"
  Demux/26 -> BusCreator/26  "TCU_Cfg Gearbox5 iBGear4"
  Demux/25 -> BusCreator/25  "TCU_Cfg Gearbox5 iBGear3"
  Demux/24 -> BusCreator/24  "TCU_Cfg Gearbox5 iBGear2"
  Demux/23 -> BusCreator/23  "TCU_Cfg Gearbox5 iBGear1"
  Demux/22 -> BusCreator/22  "TCU_Cfg Gearbox5 iBGear0"
  Demux/21 -> BusCreator/21  "TCU_Cfg Gearbox5 nBGears"
  Demux/20 -> BusCreator/20  "TCU_Cfg Gearbox5 iFGear16"
  Demux/19 -> BusCreator/19  "TCU_Cfg Gearbox5 iFGear15"
  Demux/18 -> BusCreator/18  "TCU_Cfg Gearbox5 iFGear14"
  Demux/17 -> BusCreator/17  "TCU_Cfg Gearbox5 iFGear13"
  Demux/16 -> BusCreator/16  "TCU_Cfg Gearbox5 iFGear12"
  Demux/15 -> BusCreator/15  "TCU_Cfg Gearbox5 iFGear11"
  Demux/14 -> BusCreator/14  "TCU_Cfg Gearbox5 iFGear10"
  Demux/13 -> BusCreator/13  "TCU_Cfg Gearbox5 iFGear9"
  Demux/12 -> BusCreator/12  "TCU_Cfg Gearbox5 iFGear8"
  Demux/11 -> BusCreator/11  "TCU_Cfg Gearbox5 iFGear7"
  Demux/10 -> BusCreator/10  "TCU_Cfg Gearbox5 iFGear6"
  Demux/9 -> BusCreator/9  "TCU_Cfg Gearbox5 iFGear5"
  Demux/8 -> BusCreator/8  "TCU_Cfg Gearbox5 iFGear4"
  Demux/7 -> BusCreator/7  "TCU_Cfg Gearbox5 iFGear3"
  Demux/6 -> BusCreator/6  "TCU_Cfg Gearbox5 iFGear2"
  Demux/5 -> BusCreator/5  "TCU_Cfg Gearbox5 iFGear1"
  Demux/4 -> BusCreator/4  "TCU_Cfg Gearbox5 iFGear0"
  Demux/3 -> BusCreator/3  "TCU_Cfg Gearbox5 nFGears"
  Demux/2 -> BusCreator/2  "TCU_Cfg Gearbox5 ClKind"
  Demux/1 -> BusCreator/1  "TCU_Cfg Gearbox5 GBKind"
  BusCreator/1 -> Out/1
  In/1 -> Demux/1

== system PTTransmCU/CarMaker/IPG Vehicle/PowerTrain/TCU Example/PTTransmCU_In/CreateBus TCU_Cfg Gearbox6 ==
  In : Inport
  BusCreator : BusCreator  Inputs=38
  Demux : Demux  Outputs=38
      settings: DisplayOption=none
  Out : Outport  VectorParamsAs1DForOutWhenUnconnected=off
  wires:
  Demux/38 -> BusCreator/38  "TCU_Cfg Gearbox6 iBGear16"
  Demux/37 -> BusCreator/37  "TCU_Cfg Gearbox6 iBGear15"
  Demux/36 -> BusCreator/36  "TCU_Cfg Gearbox6 iBGear14"
  Demux/35 -> BusCreator/35  "TCU_Cfg Gearbox6 iBGear13"
  Demux/34 -> BusCreator/34  "TCU_Cfg Gearbox6 iBGear12"
  Demux/33 -> BusCreator/33  "TCU_Cfg Gearbox6 iBGear11"
  Demux/32 -> BusCreator/32  "TCU_Cfg Gearbox6 iBGear10"
  Demux/31 -> BusCreator/31  "TCU_Cfg Gearbox6 iBGear9"
  Demux/30 -> BusCreator/30  "TCU_Cfg Gearbox6 iBGear8"
  Demux/29 -> BusCreator/29  "TCU_Cfg Gearbox6 iBGear7"
  Demux/28 -> BusCreator/28  "TCU_Cfg Gearbox6 iBGear6"
  Demux/27 -> BusCreator/27  "TCU_Cfg Gearbox6 iBGear5"
  Demux/26 -> BusCreator/26  "TCU_Cfg Gearbox6 iBGear4"
  Demux/25 -> BusCreator/25  "TCU_Cfg Gearbox6 iBGear3"
  Demux/24 -> BusCreator/24  "TCU_Cfg Gearbox6 iBGear2"
  Demux/23 -> BusCreator/23  "TCU_Cfg Gearbox6 iBGear1"
  Demux/22 -> BusCreator/22  "TCU_Cfg Gearbox6 iBGear0"
  Demux/21 -> BusCreator/21  "TCU_Cfg Gearbox6 nBGears"
  Demux/20 -> BusCreator/20  "TCU_Cfg Gearbox6 iFGear16"
  Demux/19 -> BusCreator/19  "TCU_Cfg Gearbox6 iFGear15"
  Demux/18 -> BusCreator/18  "TCU_Cfg Gearbox6 iFGear14"
  Demux/17 -> BusCreator/17  "TCU_Cfg Gearbox6 iFGear13"
  Demux/16 -> BusCreator/16  "TCU_Cfg Gearbox6 iFGear12"
  Demux/15 -> BusCreator/15  "TCU_Cfg Gearbox6 iFGear11"
  Demux/14 -> BusCreator/14  "TCU_Cfg Gearbox6 iFGear10"
  Demux/13 -> BusCreator/13  "TCU_Cfg Gearbox6 iFGear9"
  Demux/12 -> BusCreator/12  "TCU_Cfg Gearbox6 iFGear8"
  Demux/11 -> BusCreator/11  "TCU_Cfg Gearbox6 iFGear7"
  Demux/10 -> BusCreator/10  "TCU_Cfg Gearbox6 iFGear6"
  Demux/9 -> BusCreator/9  "TCU_Cfg Gearbox6 iFGear5"
  Demux/8 -> BusCreator/8  "TCU_Cfg Gearbox6 iFGear4"
  Demux/7 -> BusCreator/7  "TCU_Cfg Gearbox6 iFGear3"
  Demux/6 -> BusCreator/6  "TCU_Cfg Gearbox6 iFGear2"
  Demux/5 -> BusCreator/5  "TCU_Cfg Gearbox6 iFGear1"
  Demux/4 -> BusCreator/4  "TCU_Cfg Gearbox6 iFGear0"
  Demux/3 -> BusCreator/3  "TCU_Cfg Gearbox6 nFGears"
  Demux/2 -> BusCreator/2  "TCU_Cfg Gearbox6 ClKind"
  Demux/1 -> BusCreator/1  "TCU_Cfg Gearbox6 GBKind"
  BusCreator/1 -> Out/1
  In/1 -> Demux/1

== system PTTransmCU/CarMaker/IPG Vehicle/PowerTrain/TCU Example/PTTransmCU_In/CreateBus TCU_Cfg Gearbox7 ==
  In : Inport
  BusCreator : BusCreator  Inputs=38
  Demux : Demux  Outputs=38
      settings: DisplayOption=none
  Out : Outport  VectorParamsAs1DForOutWhenUnconnected=off
  wires:
  Demux/38 -> BusCreator/38  "TCU_Cfg Gearbox7 iBGear16"
  Demux/37 -> BusCreator/37  "TCU_Cfg Gearbox7 iBGear15"
  Demux/36 -> BusCreator/36  "TCU_Cfg Gearbox7 iBGear14"
  Demux/35 -> BusCreator/35  "TCU_Cfg Gearbox7 iBGear13"
  Demux/34 -> BusCreator/34  "TCU_Cfg Gearbox7 iBGear12"
  Demux/33 -> BusCreator/33  "TCU_Cfg Gearbox7 iBGear11"
  Demux/32 -> BusCreator/32  "TCU_Cfg Gearbox7 iBGear10"
  Demux/31 -> BusCreator/31  "TCU_Cfg Gearbox7 iBGear9"
  Demux/30 -> BusCreator/30  "TCU_Cfg Gearbox7 iBGear8"
  Demux/29 -> BusCreator/29  "TCU_Cfg Gearbox7 iBGear7"
  Demux/28 -> BusCreator/28  "TCU_Cfg Gearbox7 iBGear6"
  Demux/27 -> BusCreator/27  "TCU_Cfg Gearbox7 iBGear5"
  Demux/26 -> BusCreator/26  "TCU_Cfg Gearbox7 iBGear4"
  Demux/25 -> BusCreator/25  "TCU_Cfg Gearbox7 iBGear3"
  Demux/24 -> BusCreator/24  "TCU_Cfg Gearbox7 iBGear2"
  Demux/23 -> BusCreator/23  "TCU_Cfg Gearbox7 iBGear1"
  Demux/22 -> BusCreator/22  "TCU_Cfg Gearbox7 iBGear0"
  Demux/21 -> BusCreator/21  "TCU_Cfg Gearbox7 nBGears"
  Demux/20 -> BusCreator/20  "TCU_Cfg Gearbox7 iFGear16"
  Demux/19 -> BusCreator/19  "TCU_Cfg Gearbox7 iFGear15"
  Demux/18 -> BusCreator/18  "TCU_Cfg Gearbox7 iFGear14"
  Demux/17 -> BusCreator/17  "TCU_Cfg Gearbox7 iFGear13"
  Demux/16 -> BusCreator/16  "TCU_Cfg Gearbox7 iFGear12"
  Demux/15 -> BusCreator/15  "TCU_Cfg Gearbox7 iFGear11"
  Demux/14 -> BusCreator/14  "TCU_Cfg Gearbox7 iFGear10"
  Demux/13 -> BusCreator/13  "TCU_Cfg Gearbox7 iFGear9"
  Demux/12 -> BusCreator/12  "TCU_Cfg Gearbox7 iFGear8"
  Demux/11 -> BusCreator/11  "TCU_Cfg Gearbox7 iFGear7"
  Demux/10 -> BusCreator/10  "TCU_Cfg Gearbox7 iFGear6"
  Demux/9 -> BusCreator/9  "TCU_Cfg Gearbox7 iFGear5"
  Demux/8 -> BusCreator/8  "TCU_Cfg Gearbox7 iFGear4"
  Demux/7 -> BusCreator/7  "TCU_Cfg Gearbox7 iFGear3"
  Demux/6 -> BusCreator/6  "TCU_Cfg Gearbox7 iFGear2"
  Demux/5 -> BusCreator/5  "TCU_Cfg Gearbox7 iFGear1"
  Demux/4 -> BusCreator/4  "TCU_Cfg Gearbox7 iFGear0"
  Demux/3 -> BusCreator/3  "TCU_Cfg Gearbox7 nFGears"
  Demux/2 -> BusCreator/2  "TCU_Cfg Gearbox7 ClKind"
  Demux/1 -> BusCreator/1  "TCU_Cfg Gearbox7 GBKind"
  BusCreator/1 -> Out/1
  In/1 -> Demux/1

== system PTTransmCU/CarMaker/IPG Vehicle/PowerTrain/TCU Example/PTTransmCU_In/CreateBus TCU_Cfg Gearbox8 ==
  In : Inport
  BusCreator : BusCreator  Inputs=38
  Demux : Demux  Outputs=38
      settings: DisplayOption=none
  Out : Outport  VectorParamsAs1DForOutWhenUnconnected=off
  wires:
  Demux/38 -> BusCreator/38  "TCU_Cfg Gearbox8 iBGear16"
  Demux/37 -> BusCreator/37  "TCU_Cfg Gearbox8 iBGear15"
  Demux/36 -> BusCreator/36  "TCU_Cfg Gearbox8 iBGear14"
  Demux/35 -> BusCreator/35  "TCU_Cfg Gearbox8 iBGear13"
  Demux/34 -> BusCreator/34  "TCU_Cfg Gearbox8 iBGear12"
  Demux/33 -> BusCreator/33  "TCU_Cfg Gearbox8 iBGear11"
  Demux/32 -> BusCreator/32  "TCU_Cfg Gearbox8 iBGear10"
  Demux/31 -> BusCreator/31  "TCU_Cfg Gearbox8 iBGear9"
  Demux/30 -> BusCreator/30  "TCU_Cfg Gearbox8 iBGear8"
  Demux/29 -> BusCreator/29  "TCU_Cfg Gearbox8 iBGear7"
  Demux/28 -> BusCreator/28  "TCU_Cfg Gearbox8 iBGear6"
  Demux/27 -> BusCreator/27  "TCU_Cfg Gearbox8 iBGear5"
  Demux/26 -> BusCreator/26  "TCU_Cfg Gearbox8 iBGear4"
  Demux/25 -> BusCreator/25  "TCU_Cfg Gearbox8 iBGear3"
  Demux/24 -> BusCreator/24  "TCU_Cfg Gearbox8 iBGear2"
  Demux/23 -> BusCreator/23  "TCU_Cfg Gearbox8 iBGear1"
  Demux/22 -> BusCreator/22  "TCU_Cfg Gearbox8 iBGear0"
  Demux/21 -> BusCreator/21  "TCU_Cfg Gearbox8 nBGears"
  Demux/20 -> BusCreator/20  "TCU_Cfg Gearbox8 iFGear16"
  Demux/19 -> BusCreator/19  "TCU_Cfg Gearbox8 iFGear15"
  Demux/18 -> BusCreator/18  "TCU_Cfg Gearbox8 iFGear14"
  Demux/17 -> BusCreator/17  "TCU_Cfg Gearbox8 iFGear13"
  Demux/16 -> BusCreator/16  "TCU_Cfg Gearbox8 iFGear12"
  Demux/15 -> BusCreator/15  "TCU_Cfg Gearbox8 iFGear11"
  Demux/14 -> BusCreator/14  "TCU_Cfg Gearbox8 iFGear10"
  Demux/13 -> BusCreator/13  "TCU_Cfg Gearbox8 iFGear9"
  Demux/12 -> BusCreator/12  "TCU_Cfg Gearbox8 iFGear8"
  Demux/11 -> BusCreator/11  "TCU_Cfg Gearbox8 iFGear7"
  Demux/10 -> BusCreator/10  "TCU_Cfg Gearbox8 iFGear6"
  Demux/9 -> BusCreator/9  "TCU_Cfg Gearbox8 iFGear5"
  Demux/8 -> BusCreator/8  "TCU_Cfg Gearbox8 iFGear4"
  Demux/7 -> BusCreator/7  "TCU_Cfg Gearbox8 iFGear3"
  Demux/6 -> BusCreator/6  "TCU_Cfg Gearbox8 iFGear2"
  Demux/5 -> BusCreator/5  "TCU_Cfg Gearbox8 iFGear1"
  Demux/4 -> BusCreator/4  "TCU_Cfg Gearbox8 iFGear0"
  Demux/3 -> BusCreator/3  "TCU_Cfg Gearbox8 nFGears"
  Demux/2 -> BusCreator/2  "TCU_Cfg Gearbox8 ClKind"
  Demux/1 -> BusCreator/1  "TCU_Cfg Gearbox8 GBKind"
  BusCreator/1 -> Out/1
  In/1 -> Demux/1

== system PTTransmCU/CarMaker/IPG Vehicle/PowerTrain/TCU Example/PTTransmCU_In/CreateBus TCU_Cfg Gearbox9 ==
  In : Inport
  BusCreator : BusCreator  Inputs=38
  Demux : Demux  Outputs=38
      settings: DisplayOption=none
  Out : Outport  VectorParamsAs1DForOutWhenUnconnected=off
  wires:
  Demux/38 -> BusCreator/38  "TCU_Cfg Gearbox9 iBGear16"
  Demux/37 -> BusCreator/37  "TCU_Cfg Gearbox9 iBGear15"
  Demux/36 -> BusCreator/36  "TCU_Cfg Gearbox9 iBGear14"
  Demux/35 -> BusCreator/35  "TCU_Cfg Gearbox9 iBGear13"
  Demux/34 -> BusCreator/34  "TCU_Cfg Gearbox9 iBGear12"
  Demux/33 -> BusCreator/33  "TCU_Cfg Gearbox9 iBGear11"
  Demux/32 -> BusCreator/32  "TCU_Cfg Gearbox9 iBGear10"
  Demux/31 -> BusCreator/31  "TCU_Cfg Gearbox9 iBGear9"
  Demux/30 -> BusCreator/30  "TCU_Cfg Gearbox9 iBGear8"
  Demux/29 -> BusCreator/29  "TCU_Cfg Gearbox9 iBGear7"
  Demux/28 -> BusCreator/28  "TCU_Cfg Gearbox9 iBGear6"
  Demux/27 -> BusCreator/27  "TCU_Cfg Gearbox9 iBGear5"
  Demux/26 -> BusCreator/26  "TCU_Cfg Gearbox9 iBGear4"
  Demux/25 -> BusCreator/25  "TCU_Cfg Gearbox9 iBGear3"
  Demux/24 -> BusCreator/24  "TCU_Cfg Gearbox9 iBGear2"
  Demux/23 -> BusCreator/23  "TCU_Cfg Gearbox9 iBGear1"
  Demux/22 -> BusCreator/22  "TCU_Cfg Gearbox9 iBGear0"
  Demux/21 -> BusCreator/21  "TCU_Cfg Gearbox9 nBGears"
  Demux/20 -> BusCreator/20  "TCU_Cfg Gearbox9 iFGear16"
  Demux/19 -> BusCreator/19  "TCU_Cfg Gearbox9 iFGear15"
  Demux/18 -> BusCreator/18  "TCU_Cfg Gearbox9 iFGear14"
  Demux/17 -> BusCreator/17  "TCU_Cfg Gearbox9 iFGear13"
  Demux/16 -> BusCreator/16  "TCU_Cfg Gearbox9 iFGear12"
  Demux/15 -> BusCreator/15  "TCU_Cfg Gearbox9 iFGear11"
  Demux/14 -> BusCreator/14  "TCU_Cfg Gearbox9 iFGear10"
  Demux/13 -> BusCreator/13  "TCU_Cfg Gearbox9 iFGear9"
  Demux/12 -> BusCreator/12  "TCU_Cfg Gearbox9 iFGear8"
  Demux/11 -> BusCreator/11  "TCU_Cfg Gearbox9 iFGear7"
  Demux/10 -> BusCreator/10  "TCU_Cfg Gearbox9 iFGear6"
  Demux/9 -> BusCreator/9  "TCU_Cfg Gearbox9 iFGear5"
  Demux/8 -> BusCreator/8  "TCU_Cfg Gearbox9 iFGear4"
  Demux/7 -> BusCreator/7  "TCU_Cfg Gearbox9 iFGear3"
  Demux/6 -> BusCreator/6  "TCU_Cfg Gearbox9 iFGear2"
  Demux/5 -> BusCreator/5  "TCU_Cfg Gearbox9 iFGear1"
  Demux/4 -> BusCreator/4  "TCU_Cfg Gearbox9 iFGear0"
  Demux/3 -> BusCreator/3  "TCU_Cfg Gearbox9 nFGears"
  Demux/2 -> BusCreator/2  "TCU_Cfg Gearbox9 ClKind"
  Demux/1 -> BusCreator/1  "TCU_Cfg Gearbox9 GBKind"
  BusCreator/1 -> Out/1
  In/1 -> Demux/1

== system PTTransmCU/CarMaker/IPG Vehicle/PowerTrain/TCU Example/PTTransmCU_In/CreateBus TCU_Cfg Misc ==
  In : Inport
  BusCreator : BusCreator  Inputs=3
  Demux : Demux  Outputs=3
      settings: DisplayOption=none
  Out : Outport  VectorParamsAs1DForOutWhenUnconnected=off
  wires:
  Demux/2 -> BusCreator/2  "TCU_Cfg nGearbox"
  Demux/1 -> BusCreator/1  "TCU_Cfg ClKind"
  BusCreator/1 -> Out/1
  In/1 -> Demux/1
  Demux/3 -> BusCreator/3  "TCU_Cfg nClutch"

== system PTTransmCU/CarMaker/IPG Vehicle/PowerTrain/TCU Example/TCU ClutchOut/CreateBus TCU ClutchOut0 ==
  In : Inport
  BusCreator : BusCreator  Inputs=1
  Demux : Demux  Outputs=1
      settings: DisplayOption=none
  Out : Outport  VectorParamsAs1DForOutWhenUnconnected=off
  wires:
  Demux/1 -> BusCreator/1  "TCU ClutchOut0 Pos"
  BusCreator/1 -> Out/1
  In/1 -> Demux/1

== system PTTransmCU/CarMaker/IPG Vehicle/PowerTrain/TCU Example/TCU ClutchOut/CreateBus TCU ClutchOut1 ==
  In : Inport
  BusCreator : BusCreator  Inputs=1
  Demux : Demux  Outputs=1
      settings: DisplayOption=none
  Out : Outport  VectorParamsAs1DForOutWhenUnconnected=off
  wires:
  Demux/1 -> BusCreator/1  "TCU ClutchOut1 Pos"
  BusCreator/1 -> Out/1
  In/1 -> Demux/1

== system PTTransmCU/CarMaker/IPG Vehicle/PowerTrain/TCU Example/TCU ClutchOut/CreateBus TCU ClutchOut10 ==
  In : Inport
  BusCreator : BusCreator  Inputs=1
  Demux : Demux  Outputs=1
      settings: DisplayOption=none
  Out : Outport  VectorParamsAs1DForOutWhenUnconnected=off
  wires:
  Demux/1 -> BusCreator/1  "TCU ClutchOut10 Pos"
  BusCreator/1 -> Out/1
  In/1 -> Demux/1

== system PTTransmCU/CarMaker/IPG Vehicle/PowerTrain/TCU Example/TCU ClutchOut/CreateBus TCU ClutchOut11 ==
  In : Inport
  BusCreator : BusCreator  Inputs=1
  Demux : Demux  Outputs=1
      settings: DisplayOption=none
  Out : Outport  VectorParamsAs1DForOutWhenUnconnected=off
  wires:
  Demux/1 -> BusCreator/1  "TCU ClutchOut11 Pos"
  BusCreator/1 -> Out/1
  In/1 -> Demux/1

== system PTTransmCU/CarMaker/IPG Vehicle/PowerTrain/TCU Example/TCU ClutchOut/CreateBus TCU ClutchOut2 ==
  In : Inport
  BusCreator : BusCreator  Inputs=1
  Demux : Demux  Outputs=1
      settings: DisplayOption=none
  Out : Outport  VectorParamsAs1DForOutWhenUnconnected=off
  wires:
  Demux/1 -> BusCreator/1  "TCU ClutchOut2 Pos"
  BusCreator/1 -> Out/1
  In/1 -> Demux/1

== system PTTransmCU/CarMaker/IPG Vehicle/PowerTrain/TCU Example/TCU ClutchOut/CreateBus TCU ClutchOut3 ==
  In : Inport
  BusCreator : BusCreator  Inputs=1
  Demux : Demux  Outputs=1
      settings: DisplayOption=none
  Out : Outport  VectorParamsAs1DForOutWhenUnconnected=off
  wires:
  Demux/1 -> BusCreator/1  "TCU ClutchOut3 Pos"
  BusCreator/1 -> Out/1
  In/1 -> Demux/1

== system PTTransmCU/CarMaker/IPG Vehicle/PowerTrain/TCU Example/TCU ClutchOut/CreateBus TCU ClutchOut4 ==
  In : Inport
  BusCreator : BusCreator  Inputs=1
  Demux : Demux  Outputs=1
      settings: DisplayOption=none
  Out : Outport  VectorParamsAs1DForOutWhenUnconnected=off
  wires:
  Demux/1 -> BusCreator/1  "TCU ClutchOut4 Pos"
  BusCreator/1 -> Out/1
  In/1 -> Demux/1

== system PTTransmCU/CarMaker/IPG Vehicle/PowerTrain/TCU Example/TCU ClutchOut/CreateBus TCU ClutchOut5 ==
  In : Inport
  BusCreator : BusCreator  Inputs=1
  Demux : Demux  Outputs=1
      settings: DisplayOption=none
  Out : Outport  VectorParamsAs1DForOutWhenUnconnected=off
  wires:
  Demux/1 -> BusCreator/1  "TCU ClutchOut5 Pos"
  BusCreator/1 -> Out/1
  In/1 -> Demux/1

== system PTTransmCU/CarMaker/IPG Vehicle/PowerTrain/TCU Example/TCU ClutchOut/CreateBus TCU ClutchOut6 ==
  In : Inport
  BusCreator : BusCreator  Inputs=1
  Demux : Demux  Outputs=1
      settings: DisplayOption=none
  Out : Outport  VectorParamsAs1DForOutWhenUnconnected=off
  wires:
  Demux/1 -> BusCreator/1  "TCU ClutchOut6 Pos"
  BusCreator/1 -> Out/1
  In/1 -> Demux/1

== system PTTransmCU/CarMaker/IPG Vehicle/PowerTrain/TCU Example/TCU ClutchOut/CreateBus TCU ClutchOut7 ==
  In : Inport
  BusCreator : BusCreator  Inputs=1
  Demux : Demux  Outputs=1
      settings: DisplayOption=none
  Out : Outport  VectorParamsAs1DForOutWhenUnconnected=off
  wires:
  Demux/1 -> BusCreator/1  "TCU ClutchOut7 Pos"
  BusCreator/1 -> Out/1
  In/1 -> Demux/1

== system PTTransmCU/CarMaker/IPG Vehicle/PowerTrain/TCU Example/TCU ClutchOut/CreateBus TCU ClutchOut8 ==
  In : Inport
  BusCreator : BusCreator  Inputs=1
  Demux : Demux  Outputs=1
      settings: DisplayOption=none
  Out : Outport  VectorParamsAs1DForOutWhenUnconnected=off
  wires:
  Demux/1 -> BusCreator/1  "TCU ClutchOut8 Pos"
  BusCreator/1 -> Out/1
  In/1 -> Demux/1

== system PTTransmCU/CarMaker/IPG Vehicle/PowerTrain/TCU Example/TCU ClutchOut/CreateBus TCU ClutchOut9 ==
  In : Inport
  BusCreator : BusCreator  Inputs=1
  Demux : Demux  Outputs=1
      settings: DisplayOption=none
  Out : Outport  VectorParamsAs1DForOutWhenUnconnected=off
  wires:
  Demux/1 -> BusCreator/1  "TCU ClutchOut9 Pos"
  BusCreator/1 -> Out/1
  In/1 -> Demux/1

== system PTTransmCU/CarMaker/IPG Vehicle/PowerTrain/TCU Example/TCU Example/Calculate GearNoTrg ==
  GearNo : Inport
  rotvRef : Inport  Port=2
  SelectorCtrl : Inport  Port=3
  lastGearNoTrg : Inport  Port=4
  ShiftingTable : Inport  Port=5
  nFGears : Inport  Port=6
  Abs : Abs  SaturateOnIntegerOverflow=off
  Backwards : Subsystem  TreatAsAtomicUnit=on
  Bias : Bias  Bias=-1  SaturateOnIntegerOverflow=off
  Bias1 : Bias  Bias=-2  SaturateOnIntegerOverflow=off
  Constant : Constant
  Driving : Subsystem  TreatAsAtomicUnit=on
  Gain : Gain  Gain=3
  Lower Limit : MultiPortSwitch  DataPortOrder=Zero-based contiguous  Inputs=1  zeroidx=on  SaturateOnIntegerOverflow=off  InputSameDT=off
  Merge : Merge  Inputs=3
  Switch : Switch  Criteria=u2 ~= 0  SaturateOnIntegerOverflow=off  InputSameDT=off
  Switch Case : SwitchCase  CaseConditions={1,-1}
  Upper Limit : MultiPortSwitch  DataPortOrder=Zero-based contiguous  Inputs=1  zeroidx=on  SaturateOnIntegerOverflow=off  InputSameDT=off
  else : Subsystem  TreatAsAtomicUnit=on
  rpm2radsec : Gain  Gain=0.104719755
  rpm2radsec1 : Gain  Gain=0.104719755
  GearNoTrg : Outport  VectorParamsAs1DForOutWhenUnconnected=off
  wires:
  Constant/1 -> Switch/3
  Switch/1 -> Abs/1
  lastGearNoTrg/1 -> Driving/6(GearNoTrg_last)
  nFGears/1 -> Driving/5(nFGears)
  rpm2radsec1/1 -> Driving/3(Lower Limit)
  rpm2radsec/1 -> Driving/2(Upper Limit)
  rotvRef/1 -> Driving/4(rotvRef)
  Abs/1 -> Gain/1
  Switch Case/3 -> else/Action
  Switch Case/2 -> Backwards/Action
  Merge/1 -> GearNoTrg/1
  else/1(GearNoTrg) -> Merge/3
  Backwards/1(GearNoTrg) -> Merge/2
  Driving/1(GearNoTrg) -> Merge/1
  Switch Case/1 -> Driving/Action
  SelectorCtrl/1 -> Switch Case/1
  Lower Limit/1 -> rpm2radsec1/1
  GearNo/1 -> Switch/1, Switch/2, Driving/1(GearNo)
  Bias1/1 -> Lower Limit/1
  Gain/1 -> Bias1/1, Bias/1
  ShiftingTable/1 -> Lower Limit/2, Upper Limit/2
  Bias/1 -> Upper Limit/1
  Upper Limit/1 -> rpm2radsec/1

== system PTTransmCU/CarMaker/IPG Vehicle/PowerTrain/TCU Example/TCU Example/Limit GearNoTrg ==
  GearNoTrg : Inport
  nGears : Inport  Port=2
  Bus Selector : BusSelector  OutputSignals=TCU_Cfg Gearbox0 nFGears,TCU_Cfg Gearbox0 nBGears
  Gain : Gain  Gain=-1
  Saturation Dynamic : simulink/Discontinuities/Saturation Dynamic  OutMin=[]  OutMax=[]  OutDataTypeStr=Inherit: Same as second input  OutDataType=sfix(16)  OutScaling=2^-10  DoSatur=off
  GearNoTrg_limited : Outport  VectorParamsAs1DForOutWhenUnconnected=off
  wires:
  nGears/1 -> Bus Selector/1
  Saturation Dynamic/1 -> GearNoTrg_limited/1
  Gain/1 -> Saturation Dynamic/3
  Bus Selector/2 -> Gain/1  "<TCU_Cfg Gearbox0 nBGears>"
  Bus Selector/1 -> Saturation Dynamic/1  "<TCU_Cfg Gearbox0 nFGears>"
  GearNoTrg/1 -> Saturation Dynamic/2

== system PTTransmCU/CarMaker/IPG Vehicle/PowerTrain/TCU Example/TCU Example/Retrun Zero ==
  Bus Creator : BusCreator  Inputs=2
  Constant : Constant  Value=0
  Constant1 : Constant  Value=0
  GearBoxOut : Outport  VectorParamsAs1DForOutWhenUnconnected=off
  wires:
  Bus Creator/1 -> GearBoxOut/1
  Constant1/1 -> Bus Creator/2  "TCU GearBoxIn set_ParkBrake"
  Constant/1 -> Bus Creator/1  "TCU GearBoxIn GearNoTrg"
